simulink model "IM_SpeedController_Design"  (R2024b)
settings: Solver=VariableStepAuto  StartTime=0.0  StopTime=2  RelTol=1e-3
undefined symbols (not defined in the file): ctrl, J, lambda_Rd_ref, Lm, Lr, p, Ts
libraries: cstblocks x5
settings Model: Creator=overflow  LastModifiedBy=matth

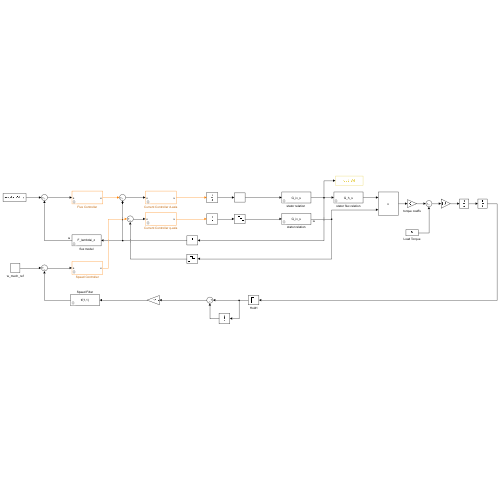
[thumbnail: Simulink's stored preview of the top-level diagram]
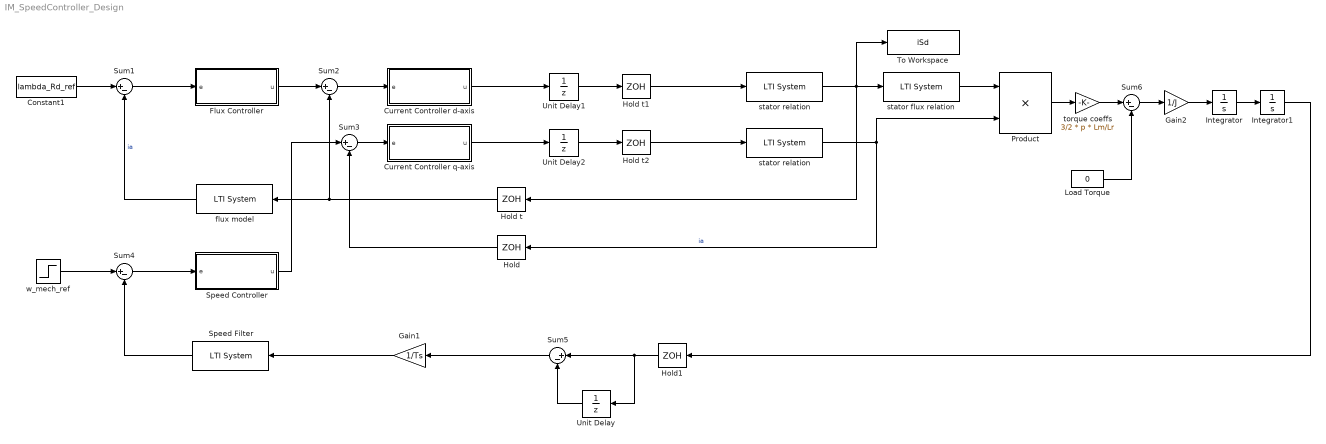
== system IM_SpeedController_Design ==
  " Hold" : ZeroOrderHold  SampleTime=-1
  " Hold t" : ZeroOrderHold  SampleTime=-1
  " Hold t1" : ZeroOrderHold  SampleTime=-1
  " Hold t2" : ZeroOrderHold  SampleTime=-1
  " Hold1" : ZeroOrderHold  SampleTime=-1
  Constant1 : Constant  Value=lambda_Rd_ref
  Current Controller d-axis : Subsystem  mask{ctrl=ctrl.i}
      mask prompts: ctrl "Controller Struct"
  Current Controller q-axis : Subsystem  mask{ctrl=ctrl.i}
      mask prompts: ctrl "Controller Struct"
  Flux Controller : Subsystem  mask{ctrl=ctrl.lambda}
      mask prompts: ctrl "Controller Struct"
  Gain1 : Gain  Gain=1/Ts
  Gain2 : Gain  Gain=1/J
  Integrator : Integrator
  Integrator1 : Integrator
  Load Torque : Constant  Value=0
  Product : Product
  Speed Controller : Subsystem  mask{ctrl=ctrl.omega}
      mask prompts: ctrl "Controller Struct"
  Speed Filter : cstblocks/LTI System  sys=tf(1,1)  IC=[]  PadeOrder=0
      link override Internal: InitialCondition=w_start
  Sum{1..6} (6 alike) : Sum  Inputs=|+-
  To Workspace : ToWorkspace  VariableName=iSd  SaveFormat=Timeseries  SampleTime=-1
  Unit Delay : UnitDelay  SampleTime=-1  HasFrameUpgradeWarning=on
  Unit Delay1 : UnitDelay  SampleTime=-1  HasFrameUpgradeWarning=on
  Unit Delay2 : UnitDelay  SampleTime=-1  HasFrameUpgradeWarning=on
  flux model : cstblocks/LTI System  sys=F_lambdai_z  IC=[0]  PadeOrder=0
  stator flux relation : cstblocks/LTI System  sys=G_h_s  IC=[0]  PadeOrder=0
  stator relation : cstblocks/LTI System  sys=G_iv_s  IC=[0]  PadeOrder=0
  "stator relation " : cstblocks/LTI System  sys=G_iv_s  IC=[0]  PadeOrder=0
  torque coeffs : Gain  Gain=3/2 * p * Lm/Lr
  w_mech_ref : Step  Time=0  SampleTime=0
  wires:
  Sum1/1 -> Flux Controller/1(e)
  Flux Controller/1(u) -> Sum2/1
  Sum2/1 -> Current Controller d-axis/1(e)
  Sum3/1 -> Current Controller q-axis/1(e)
  Speed Controller/1(u) -> Sum3/1
  Sum4/1 -> Speed Controller/1(e)
  flux model/1 -> Sum1/2  "ia"
  " Hold t"/1 -> Sum2/2, flux model/1
  Current Controller d-axis/1(u) -> Unit Delay1/1
  " Hold t1"/1 -> "stator relation "/1
  " Hold t2"/1 -> stator relation/1
  Current Controller q-axis/1(u) -> Unit Delay2/1
  " Hold"/1 -> Sum3/2
  "stator relation "/1 -> To Workspace/1, " Hold t"/1, stator flux relation/1
  stator relation/1 -> Product/2, " Hold"/1  "ia"
  Speed Filter/1 -> Sum4/2
  Unit Delay/1 -> Sum5/2
  " Hold1"/1 -> Unit Delay/1, Sum5/1
  Sum5/1 -> Gain1/1
  Integrator1/1 -> " Hold1"/1
  Load Torque/1 -> Sum6/2
  stator flux relation/1 -> Product/1
  Product/1 -> torque coeffs/1
  torque coeffs/1 -> Sum6/1
  Sum6/1 -> Gain2/1
  Integrator/1 -> Integrator1/1
  Gain2/1 -> Integrator/1
  Gain1/1 -> Speed Filter/1
  Unit Delay2/1 -> " Hold t2"/1
  Unit Delay1/1 -> " Hold t1"/1
  Constant1/1 -> Sum1/1
  w_mech_ref/1 -> Sum4/1

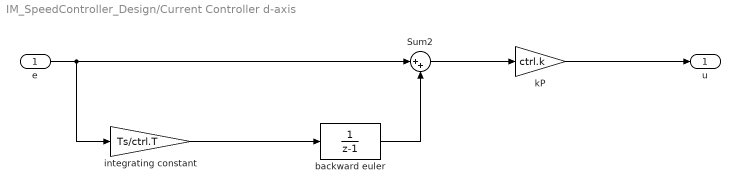
== system IM_SpeedController_Design/Current Controller d-axis ==
  e : Inport
  Sum2 : Sum  Inputs=|++
  backward euler : DiscreteTransferFcn  Denominator=[1 -1]
  integrating constant : Gain  Gain=Ts/ctrl.T
  kP : Gain  Gain=ctrl.k
  u : Outport
  wires:
  backward euler/1 -> Sum2/2
  kP/1 -> u/1
  Sum2/1 -> kP/1
  e/1 -> Sum2/1, integrating constant/1
  integrating constant/1 -> backward euler/1

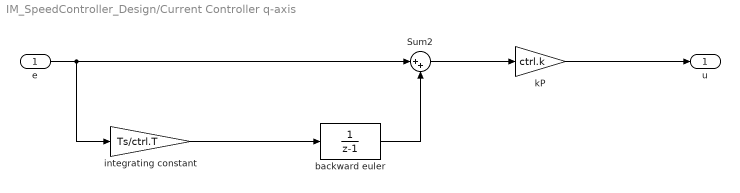
== system IM_SpeedController_Design/Current Controller q-axis ==
  e : Inport
  Sum2 : Sum  Inputs=|++
  backward euler : DiscreteTransferFcn  Denominator=[1 -1]
  integrating constant : Gain  Gain=Ts/ctrl.T
  kP : Gain  Gain=ctrl.k
  u : Outport
  wires:
  backward euler/1 -> Sum2/2
  kP/1 -> u/1
  Sum2/1 -> kP/1
  e/1 -> Sum2/1, integrating constant/1
  integrating constant/1 -> backward euler/1

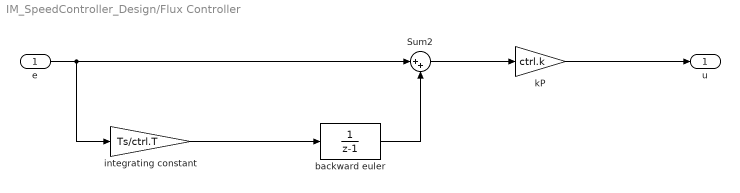
== system IM_SpeedController_Design/Flux Controller ==
  e : Inport
  Sum2 : Sum  Inputs=|++
  backward euler : DiscreteTransferFcn  Denominator=[1 -1]
  integrating constant : Gain  Gain=Ts/ctrl.T
  kP : Gain  Gain=ctrl.k
  u : Outport
  wires:
  backward euler/1 -> Sum2/2
  kP/1 -> u/1
  Sum2/1 -> kP/1
  e/1 -> Sum2/1, integrating constant/1
  integrating constant/1 -> backward euler/1

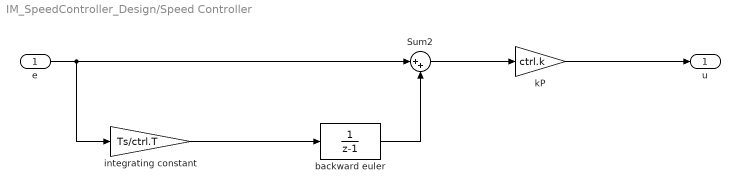
== system IM_SpeedController_Design/Speed Controller ==
  e : Inport
  Sum2 : Sum  Inputs=|++
  backward euler : DiscreteTransferFcn  Denominator=[1 -1]
  integrating constant : Gain  Gain=Ts/ctrl.T
  kP : Gain  Gain=ctrl.k
  u : Outport
  wires:
  backward euler/1 -> Sum2/2
  kP/1 -> u/1
  Sum2/1 -> kP/1
  e/1 -> Sum2/1, integrating constant/1
  integrating constant/1 -> backward euler/1
